simulink model "convType_ClosedLoop_delay_continousPlant_2018a"  (R2018a)
settings: Solver=VariableStepAuto  StartTime=0.0  StopTime=10.0  RelTol=1e-3
settings Model: Creator=dell-wi  LastModifiedBy=dell-wi

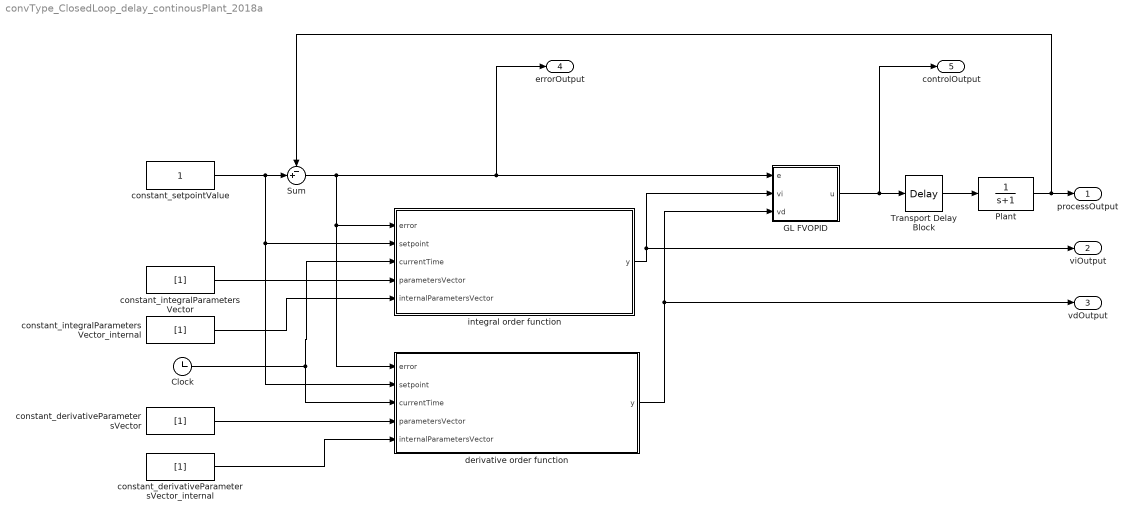
== system convType_ClosedLoop_delay_continousPlant_2018a ==
  Clock : Clock
  GL FVOPID : Subsystem  mask{kp=1, ki=1, kd=0, sampleTime=1, inputBufferSize=-1, constantIntegralOrder=1, constantDerivativeOrder=1, satEnab=off, satHigh=inf, satLow=-inf}
      mask prompts: kp "Proportional (P)"; ki "Integral (I)"; kd "Derivative (D)"; sampleTime "Sample time"; inputBufferSize "Input buffer size (-1 for automatically calculated)"; constantIntegralOrder "Integral order"; constantDerivativeOrder "Derivative order"; satEnab "Limit output"; satHigh "Upper limit"; satLow "Lower limit"
      mask init:
      | % Initialize block parameters
      | fvopidToolbox.library.utils.initializeBasicModelParameters(sampleTime, inputBufferSize,'fvopidConv');
      settings: CopyFcn=set_param(gcbh, 'LinkStatus', 'none');
      mask Callback satEnab:
      | limitOutputCheckBoxValue = get_param(gcb,'satEnab');
      | if strcmp(limitOutputCheckBoxValue, 'on')
      |    fvopidToolbox.library.utils.setMaskParameterPropertyValue('satHigh', 'MaskEnables', 'on');
      |    fvopidToolbox.library.utils.setMaskParameterPropertyValue('satLow', 'MaskEnables', 'on');
      | else
      |    fvopidToolbox.library.utils.setMaskParameterPropertyValue('satHigh', 'MaskEnables', 'off');
      |    fvopidToolbox.library.utils.setMaskParameterPropertyValue('satLow', 'MaskEnables', 'off');
      | end
      mask DialogControl mainTab Prompt: Main
      mask DialogControl controllerParametersGroupBox Prompt: Controller parameters
      mask DialogControl outputSaturationTab Prompt: Output saturation
      mask DialogControl outputSaturationGroupBox Prompt: Output saturation
  Plant : TransferFcn  Denominator="[1  1]"
  Sum : Sum  Inputs=-+|
  Transport Delay Block : TransportDelay
  constant_derivativeParametersVector : Constant  Value=[1]
  constant_derivativeParametersVector_internal : Constant  Value=[1]
  constant_integralParametersVector : Constant  Value=[1]
  constant_integralParametersVector_internal : Constant  Value=[1]
  constant_setpointValue : Constant
  derivative order function : MATLAB Function  TreatAsAtomicUnit=on
  integral order function : MATLAB Function  TreatAsAtomicUnit=on
  processOutput : Outport  SampleTime=0.01
  viOutput : Outport  Port=2  SampleTime=0.01
  vdOutput : Outport  Port=3  SampleTime=0.01
  errorOutput : Outport  Port=4  SampleTime=0.01
  controlOutput : Outport  Port=5  SampleTime=0.01
  wires:
  Sum/1 -> derivative order function/1(error), integral order function/1(error), GL FVOPID/1(e), errorOutput/1
  constant_setpointValue/1 -> derivative order function/2(setpoint), integral order function/2(setpoint), Sum/2
  Plant/1 -> processOutput/1, Sum/1
  GL FVOPID/1(u) -> controlOutput/1, Transport Delay Block/1
  integral order function/1(y) -> GL FVOPID/2(vi), viOutput/1
  derivative order function/1(y) -> GL FVOPID/3(vd), vdOutput/1
  constant_integralParametersVector/1 -> integral order function/4(parametersVector)
  constant_derivativeParametersVector/1 -> derivative order function/4(parametersVector)
  Clock/1 -> integral order function/3(currentTime), derivative order function/3(currentTime)
  constant_derivativeParametersVector_internal/1 -> derivative order function/5(internalParametersVector)
  constant_integralParametersVector_internal/1 -> integral order function/5(internalParametersVector)
  Transport Delay Block/1 -> Plant/1

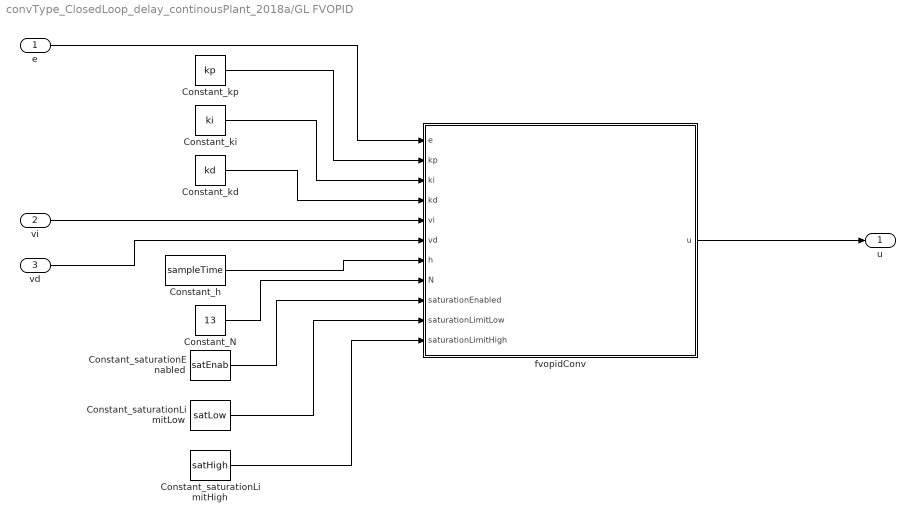
== system convType_ClosedLoop_delay_continousPlant_2018a/GL FVOPID ==
  e : Inport
  vi : Inport  Port=2
  vd : Inport  Port=3
  Constant_N : Constant  Value=13
  Constant_h : Constant  Value=sampleTime
  Constant_kd : Constant  Value=kd
  Constant_ki : Constant  Value=ki
  Constant_kp : Constant  Value=kp
  Constant_saturationEnabled : Constant  Value=satEnab
  Constant_saturationLimitHigh : Constant  Value=satHigh
  Constant_saturationLimitLow : Constant  Value=satLow
  fvopidConv : MATLAB Function  TreatAsAtomicUnit=on  SystemSampleTime=1
  u : Outport
  wires:
  Constant_saturationLimitHigh/1 -> fvopidConv/11(saturationLimitHigh)
  e/1 -> fvopidConv/1(e)
  Constant_N/1 -> fvopidConv/8(N)
  Constant_h/1 -> fvopidConv/7(h)
  Constant_kp/1 -> fvopidConv/2(kp)
  Constant_saturationLimitLow/1 -> fvopidConv/10(saturationLimitLow)
  fvopidConv/1(u) -> u/1
  Constant_saturationEnabled/1 -> fvopidConv/9(saturationEnabled)
  Constant_kd/1 -> fvopidConv/4(kd)
  Constant_ki/1 -> fvopidConv/3(ki)
  vi/1 -> fvopidConv/5(vi)
  vd/1 -> fvopidConv/6(vd)

== matlab function convType_ClosedLoop_delay_continousPlant_2018a/derivative order function ==
  data: error input; y output; setpoint input; currentTime input; parametersVector input; internalParametersVector input
function y = derivativeOrderFunction(error, setpoint, currentTime, parametersVector, internalParametersVector)
y = parametersVector(1);

== matlab function convType_ClosedLoop_delay_continousPlant_2018a/integral order function ==
  data: error input; y output; setpoint input; currentTime input; parametersVector input; internalParametersVector input
function y = integralOrderFunction(error, setpoint, currentTime, parametersVector, internalParametersVector)
y = parametersVector(1);

== matlab function convType_ClosedLoop_delay_continousPlant_2018a/GL FVOPID/fvopidConv ==
  data: e input; u output; kp input; ki input; kd input; vi input; vd input; h input; N input; saturationEnabled input; saturationLimitLow input; saturationLimitHigh input
function u = fvopidConv(e, kp, ki, kd, vi, vd, h, N, saturationEnabled, saturationLimitLow, saturationLimitHigh)
    u = fvopidToolbox.fvopid.fvopidConv(e, kp, ki, kd, vi, vd, h, N, saturationEnabled, saturationLimitLow, saturationLimitHigh);
